simulink model "sstdr_basic"  (R2024b)
settings: Solver=ode45  StartTime=0.0  StopTime=0.00025575  FixedStep=5e-9  MaxStep=1.5625e-09  RelTol=1e-3
undefined symbols (not defined in the file): sim_max_step, sim_ts
libraries: spsDistributedParametersLineFrequencyDependentLib x15, spsGroundLib x6, spsSeriesRLCBranchLib x4, spsVoltageMeasurementLib x2, spsControlledVoltageSourceLib x1, spspowerguiLib x1
settings Model: Creator=nathanielfargo  LastModifiedBy=nathanielfargo

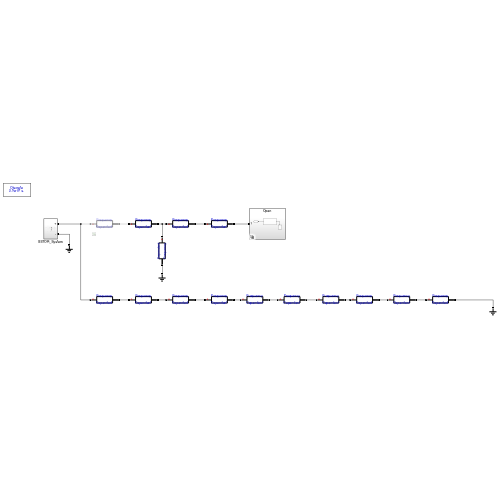
[thumbnail: Simulink's stored preview of the top-level diagram]
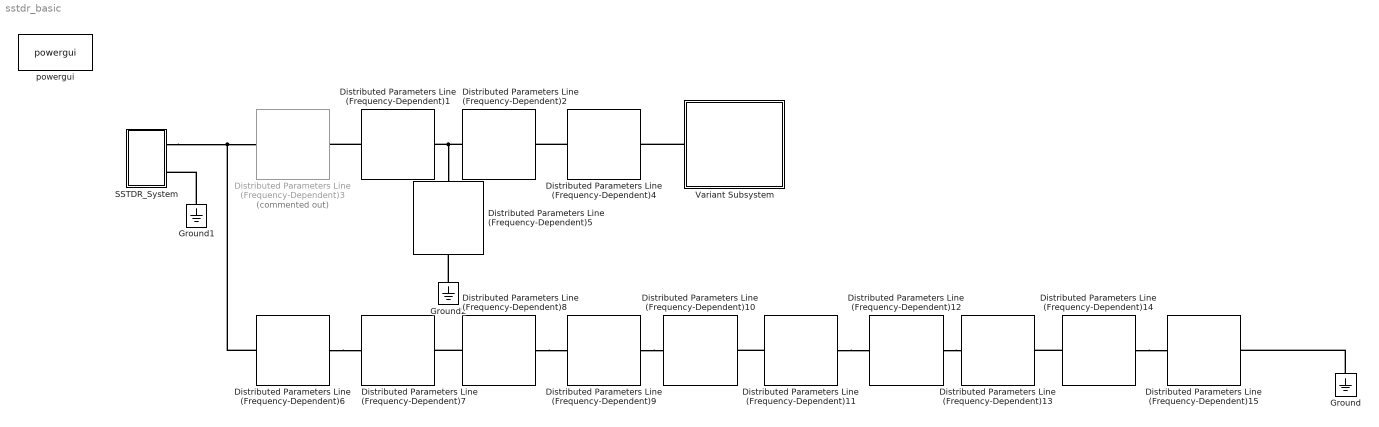
== system sstdr_basic ==
  Distributed Parameters Line (Frequency-Dependent){1..2,4..15} (14 alike) : spsDistributedParametersLineFrequencyDependentLib/Distributed Parameters Line (Frequency-Dependent)  WBfile=./config/line_params/line_test.mat  L=1  NbPhases=1  Frange=1.00e+00 Hz to 1.00e+09 Hz, 141 points.  Comments=|  Measurements=None
      | Example of a 735 KV three-phase line
      |
      | Three bundles of 4 Bersfort ACSR 1355 MCM conductors
      | Two 1/2 inch diameter steel grounds wires
      |
      | Ytower =Ymin =  average heights of conductors
      settings: LibrarySourceBlock=|
      | sps_lib/Power Grid Elements/Distributed Parameters Line
      | (Frequency-Dependent)
  Distributed Parameters Line (Frequency-Dependent)3 : spsDistributedParametersLineFrequencyDependentLib/Distributed Parameters Line (Frequency-Dependent)  Commented=on  WBfile=./config/line_params/line_test.mat  L=1  NbPhases=1  Frange=1.00e+00 Hz to 1.00e+09 Hz, 141 points.  Comments=|  Measurements=None
      | Example of a 735 KV three-phase line
      |
      | Three bundles of 4 Bersfort ACSR 1355 MCM conductors
      | Two 1/2 inch diameter steel grounds wires
      |
      | Ytower =Ymin =  average heights of conductors
      settings: LibrarySourceBlock=|
      | sps_lib/Power Grid Elements/Distributed Parameters Line
      | (Frequency-Dependent)
  Ground : spsGroundLib/Ground  LConnTagsString=a
  Ground1 : spsGroundLib/Ground  LConnTagsString=a
  Ground2 : spsGroundLib/Ground  LConnTagsString=a
  SSTDR_System : Subsystem
  Variant Subsystem : Subsystem  Variant=on  VariantControlMode=label  LabelModeActiveChoice=Open
  powergui : spspowerguiLib/powergui  Priority=1  SimulationMode=Discrete  SampleTime=sim_max_step  frequency=60  Iterations=50  frequencyindice=0  Pbase=100e6  ErrMax=1e-4  UnitsV=kV  UnitsW=MW  buscounter=0  FunctionMessages=off  echomessages=off  EnableUseOfTLC=off  CurrentSourceSwitches=off  DisableSnubberDevices=off  DisableRonSwitches=off  DisableVfSwitches=off  DisplayEquations=off  AutomaticDiscreteSolvers=off  SolverType=Tustin/Backward Euler (TBE)  Interpol=off  ExternalGateDelay=off  methode=off  Ts=100  x0status=blocks  SPID=on  SwTol=0  HookPort=off  NonlinearTolerance=1e-4  nMaxIteration=100  ContinueOnMaxIteration=off  RestoreLinks=warning  ResistiveCurrentMeasurement=off  Frange=[0:2:500]  Ylog=off  Xlog=on  ShowGrid=off  save=off  variable=ZData  structure=0  ZoomFFT=off  StartTime=0.0  cycles=1  DisplayStyle=1  fundamental=60  FreqAxis=off  MaxFrequency=1000  frequencyindicesteady=1  RmsSteady=1  display=off
  connections:
  Variant Subsystem/LConn1 -- Distributed Parameters Line (Frequency-Dependent)4/RConn1
  Distributed Parameters Line (Frequency-Dependent)1/LConn1 -- Distributed Parameters Line (Frequency-Dependent)3/RConn1
  Distributed Parameters Line (Frequency-Dependent)2/LConn1 -- Distributed Parameters Line (Frequency-Dependent)5/LConn1 -- Distributed Parameters Line (Frequency-Dependent)1/RConn1
  Distributed Parameters Line (Frequency-Dependent)4/LConn1 -- Distributed Parameters Line (Frequency-Dependent)2/RConn1
  Ground2/LConn1 -- Distributed Parameters Line (Frequency-Dependent)5/RConn1
  SSTDR_System/RConn1 -- Distributed Parameters Line (Frequency-Dependent)6/LConn1 -- Distributed Parameters Line (Frequency-Dependent)3/LConn1
  Ground/LConn1 -- Distributed Parameters Line (Frequency-Dependent)15/RConn1
  Ground1/LConn1 -- SSTDR_System/RConn2
  Distributed Parameters Line (Frequency-Dependent)6/RConn1 -- Distributed Parameters Line (Frequency-Dependent)7/LConn1
  Distributed Parameters Line (Frequency-Dependent)8/RConn1 -- Distributed Parameters Line (Frequency-Dependent)9/LConn1
  Distributed Parameters Line (Frequency-Dependent)8/LConn1 -- Distributed Parameters Line (Frequency-Dependent)7/RConn1
  Distributed Parameters Line (Frequency-Dependent)11/LConn1 -- Distributed Parameters Line (Frequency-Dependent)10/RConn1
  Distributed Parameters Line (Frequency-Dependent)11/RConn1 -- Distributed Parameters Line (Frequency-Dependent)12/LConn1
  Distributed Parameters Line (Frequency-Dependent)9/RConn1 -- Distributed Parameters Line (Frequency-Dependent)10/LConn1
  Distributed Parameters Line (Frequency-Dependent)14/LConn1 -- Distributed Parameters Line (Frequency-Dependent)13/RConn1
  Distributed Parameters Line (Frequency-Dependent)14/RConn1 -- Distributed Parameters Line (Frequency-Dependent)15/LConn1
  Distributed Parameters Line (Frequency-Dependent)12/RConn1 -- Distributed Parameters Line (Frequency-Dependent)13/LConn1

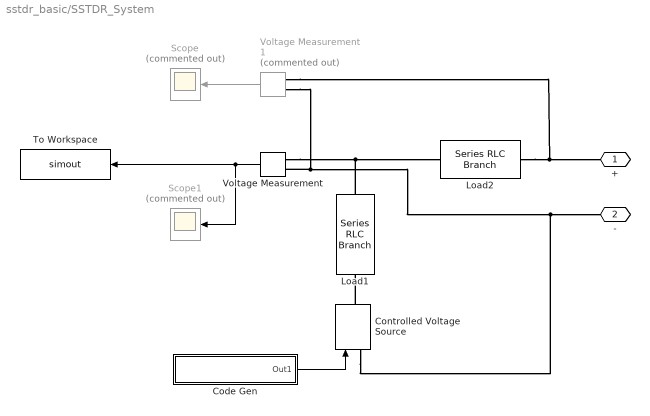
== system sstdr_basic/SSTDR_System ==
  Code Gen : Subsystem
  Controlled Voltage Source : spsControlledVoltageSourceLib/Controlled Voltage Source  Initialize=on  Source_Type=DC  Amplitude=0  Phase=0  Frequency=0  Measurements=None
  Load1 : spsSeriesRLCBranchLib/Series RLC Branch  LConnTagsString=__new0  RConnTagsString=__new0  BranchType=L  Resistance=25  Inductance=100e-6  SetiL0=off  InitialCurrent=0  Capacitance=1e-6  Setx0=off  InitialVoltage=0  Measurements=None
  Load2 : spsSeriesRLCBranchLib/Series RLC Branch  LConnTagsString=__new0  RConnTagsString=__new0  BranchType=C  Resistance=0  Inductance=0  SetiL0=off  InitialCurrent=0  Capacitance=1e-6  Setx0=off  InitialVoltage=0  Measurements=None
  Scope : Scope  Commented=on
  Scope1 : Scope  Commented=on
  To Workspace : ToWorkspace  VariableName=simout  SaveFormat=Structure With Time  SampleTime=sim_ts
  Voltage Measurement : spsVoltageMeasurementLib/Voltage Measurement  PhasorSimulation=off  OutputType=Complex  PSBequivalent=0
  Voltage Measurement1 : spsVoltageMeasurementLib/Voltage Measurement  Commented=on  PhasorSimulation=off  OutputType=Complex  PSBequivalent=0
  + : PMIOPort  Side=Right
  - : PMIOPort  Port=2  Side=Right
  wires:
  Code Gen/1(Out1) -> Controlled Voltage Source/1
  Voltage Measurement/1 -> Scope1/1, To Workspace/1
  Voltage Measurement1/1 -> Scope/1
  connections:
  Controlled Voltage Source/RConn1 -- Load1/LConn1
  Voltage Measurement/LConn1 -- Load1/RConn1 -- Load2/LConn1
  Voltage Measurement/LConn2 -- Controlled Voltage Source/LConn1 -- -/RConn1 -- Voltage Measurement1/LConn2
  Load2/RConn1 -- Voltage Measurement1/LConn1 -- +/RConn1

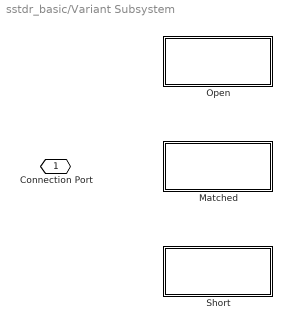
== system sstdr_basic/Variant Subsystem ==
  Matched : Subsystem  VariantControl=Matched
  Open : Subsystem  VariantControl=Open
  Short : Subsystem  VariantControl=Short
  Connection Port : PMIOPort  Side=Left

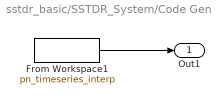
== system sstdr_basic/SSTDR_System/Code Gen ==
  From Workspace1 : FromWorkspace  VariableName=pn_timeseries_interp  OutputAfterFinalValue=Setting to zero
  Out1 : Outport
  wires:
  From Workspace1/1 -> Out1/1

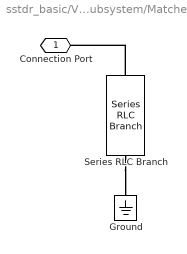
== system sstdr_basic/Variant Subsystem/Matched ==
  Ground : spsGroundLib/Ground  LConnTagsString=a
  Series RLC Branch : spsSeriesRLCBranchLib/Series RLC Branch  LConnTagsString=__new0  RConnTagsString=__new0  BranchType=RLC  Resistance=50  Inductance=0  SetiL0=off  InitialCurrent=0  Capacitance=0  Setx0=off  InitialVoltage=0  Measurements=None
  Connection Port : PMIOPort  Side=Left
  connections:
  Series RLC Branch/LConn1 -- Connection Port/RConn1
  Series RLC Branch/RConn1 -- Ground/LConn1

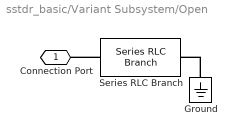
== system sstdr_basic/Variant Subsystem/Open ==
  Ground : spsGroundLib/Ground  LConnTagsString=a
  Series RLC Branch : spsSeriesRLCBranchLib/Series RLC Branch  LConnTagsString=__new0  RConnTagsString=__new0  BranchType=RLC  Resistance=10000000  Inductance=0  SetiL0=off  InitialCurrent=0  Capacitance=0  Setx0=off  InitialVoltage=0  Measurements=None
  Connection Port : PMIOPort  Side=Left
  connections:
  Series RLC Branch/LConn1 -- Connection Port/RConn1
  Ground/LConn1 -- Series RLC Branch/RConn1

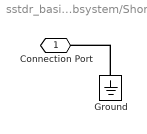
== system sstdr_basic/Variant Subsystem/Short ==
  Ground : spsGroundLib/Ground  LConnTagsString=a
  Connection Port : PMIOPort  Side=Left
  connections:
  Ground/LConn1 -- Connection Port/RConn1
